simulink model "circuitoRLCserie_v2_variablesfase"  (Simulink 5.0)
settings: Solver=ode15s  StartTime=0.0  StopTime=0.08  RelTol=1e-3
values from neighbouring files (symbols this model uses):
  C = 100e-6    (= 0.0001)    [circuitoRLCserie_valores.m]
  L = 0.05    [circuitoRLCserie_valores.m]
  R = 5    [circuitoRLCserie_valores.m]
settings Model: LastModifiedBy=gaby

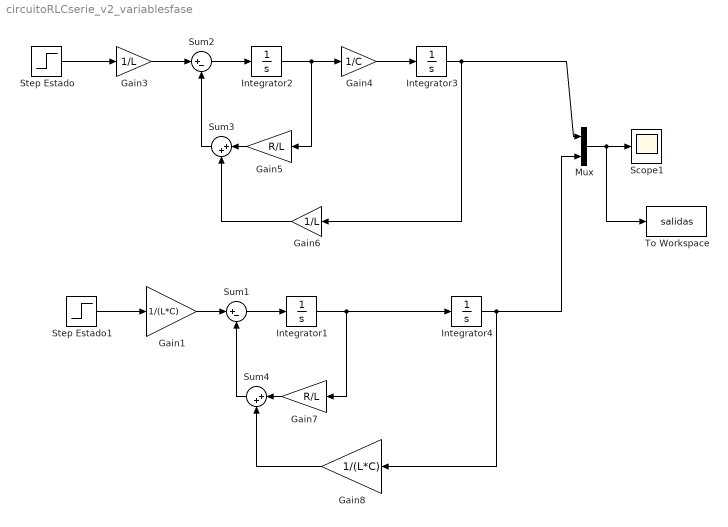
== system circuitoRLCserie_v2_variablesfase ==
  Gain1 : Gain  Gain=1/(L*C)  SaturateOnIntegerOverflow=on
  Gain3 : Gain  Gain=1/L  SaturateOnIntegerOverflow=on
  Gain4 : Gain  Gain=1/C  SaturateOnIntegerOverflow=on
  Gain5 : Gain  Orientation=left  Gain=R/L  SaturateOnIntegerOverflow=on
  Gain6 : Gain  Orientation=left  Gain=1/L  SaturateOnIntegerOverflow=on
  Gain7 : Gain  Orientation=left  Gain=R/L  SaturateOnIntegerOverflow=on
  Gain8 : Gain  Orientation=left  Gain=1/(L*C)  SaturateOnIntegerOverflow=on
  Integrator{1..4} (4 alike) : Integrator
  Mux : Mux  Inputs=2
  Scope1 : Scope
  Step Estado : Step  Time=0.002  SampleTime=0
  Step Estado1 : Step  Time=0.003  SampleTime=0
  Sum1 : Sum  Inputs=|+-  SaturateOnIntegerOverflow=on
  Sum2 : Sum  Inputs=|+-  SaturateOnIntegerOverflow=on
  Sum3 : Sum  Orientation=left  Inputs=|++  SaturateOnIntegerOverflow=on
  Sum4 : Sum  Orientation=left  Inputs=|++  SaturateOnIntegerOverflow=on
  To Workspace : ToWorkspace  VariableName=salidas  SampleTime=-1  SaveFormat=Array
  wires:
  Step Estado/1 -> Gain3/1
  Gain3/1 -> Sum2/1
  Sum2/1 -> Integrator2/1
  Integrator2/1 -> Gain4/1, Gain5/1
  Gain4/1 -> Integrator3/1
  Gain5/1 -> Sum3/1
  Gain6/1 -> Sum3/2
  Sum3/1 -> Sum2/2
  Integrator3/1 -> Gain6/1, Mux/1
  Mux/1 -> Scope1/1, To Workspace/1
  Step Estado1/1 -> Gain1/1
  Gain1/1 -> Sum1/1
  Sum1/1 -> Integrator1/1
  Integrator1/1 -> Gain7/1, Integrator4/1
  Gain7/1 -> Sum4/1
  Gain8/1 -> Sum4/2
  Sum4/1 -> Sum1/2
  Integrator4/1 -> Gain8/1, Mux/2
